simulink model "speed_controller_2017b"  (R2017b)
settings: Solver=VariableStepAuto  StartTime=0.0  StopTime=10.0  RelTol=1e-3
libraries: speedgoatlib_IO101 x2, speedgoatlib_IO106 x2, slrtlib x2
settings Model: Creator=manaka  LastModifiedBy=manaka
settings DataIOCC: ReturnWorkspaceOutputs=on
settings DebuggingCC: UnconnectedInputMsg=none  UnconnectedOutputMsg=none  UnconnectedLineMsg=none
settings ModelReferenceCC: EnableRefExpFcnMdlSchedulingChecks=off
settings SFSimCC: SimUseLocalCustomCode=on
settings RTWCC: Description=Generic Real-Time Target  RTWUseLocalCustomCode=on

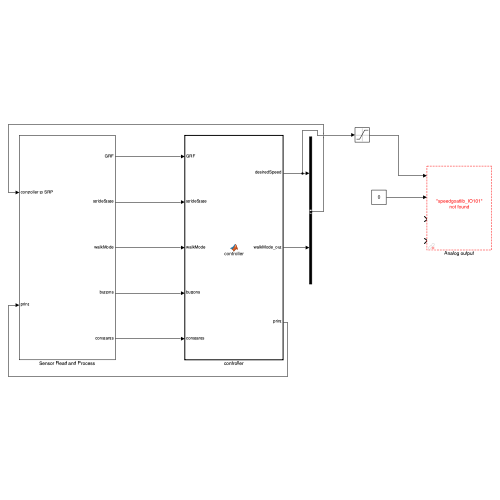
[thumbnail: Simulink's stored preview of the top-level diagram]
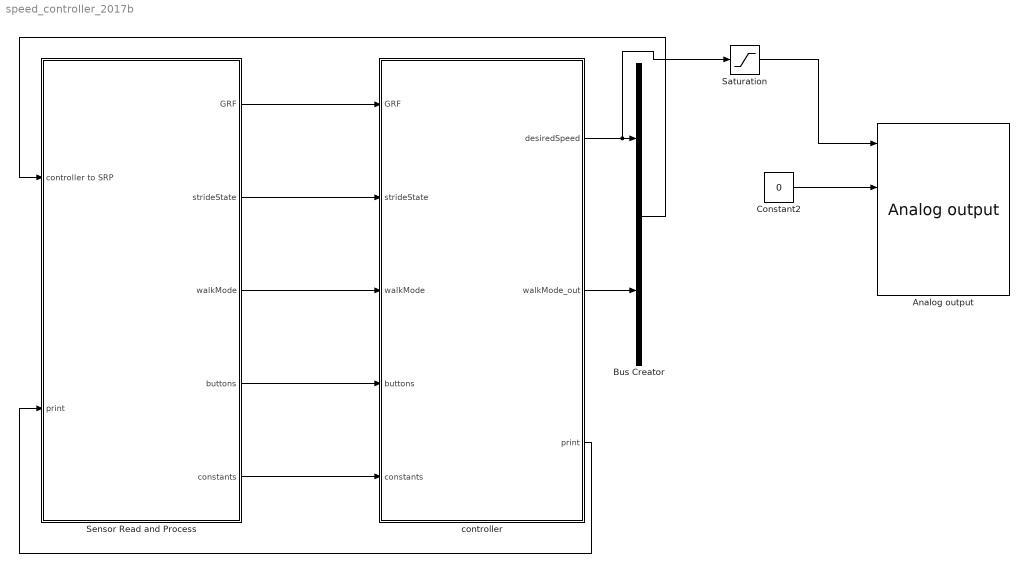
== system speed_controller_2017b ==
  Analog output : speedgoatlib_IO101/Analog output  id=1  channel=[1,2,3,4]  reset=[1,1,1,1]  initValue=[0,0,0,0]  ts=0.001  pciSlot=-1
  Bus Creator : BusCreator  Inputs=2
  Constant2 : Constant  Value=0
  Saturation : Saturate  UpperLimit=1  LowerLimit=-1
  Sensor Read and Process : Subsystem
  controller : MATLAB Function  TreatAsAtomicUnit=on
  wires:
  Sensor Read and Process/1(GRF) -> controller/1(GRF)
  Sensor Read and Process/2(strideState) -> controller/2(strideState)
  Sensor Read and Process/3(walkMode) -> controller/3(walkMode)
  Sensor Read and Process/4(buttons) -> controller/4(buttons)
  Sensor Read and Process/5(constants) -> controller/5(constants)
  Bus Creator/1 -> Sensor Read and Process/1(controller to SRP)
  controller/1(desiredSpeed) -> Saturation/1, Bus Creator/1
  controller/2(walkMode_out) -> Bus Creator/2
  controller/3(print) -> Sensor Read and Process/2(print)
  Saturation/1 -> Analog output/1
  Constant2/1 -> Analog output/2

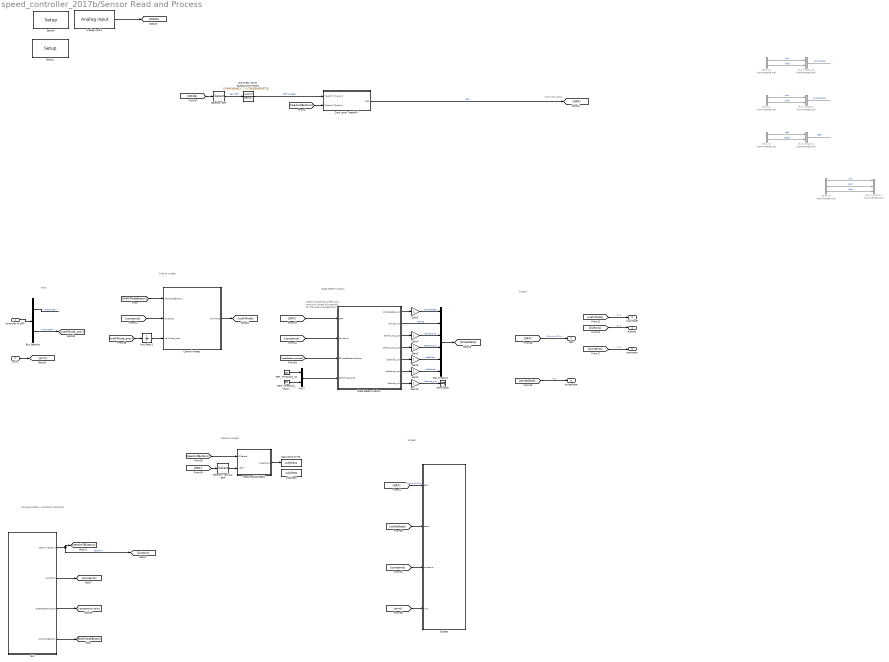
== system speed_controller_2017b/Sensor Read and Process ==
  note: Control modes
  note: Scopes
  note: Check thresholds of GRF and max/min values of threshold for stance/swing detection!
  note: State Determination
  note: GUI parameters, constants
      | & Buttons
  note: [N or Nm] 12x1
  note: Input
  note: Output
  note: Measure Weight
  controller to SRP : Inport
  print : Inport  Port=2
  "3rd Order, 25 Hz Butterworth Filter1" : DiscreteFilter  Numerator="[0.000416546139075769\t0.00124963841722731\t0.00124963841722731\t0.000416546139075769]"  Denominator="[1\t-2.68615739654814\t2.41965511096647\t-0.730165345305723]"
  Analog input3 : speedgoatlib_IO106/Analog input  id=1  channels=20  range=1  coupling=1  ts=dt  initiator=1  pciSlot=-1
  Bus Creator1 : BusCreator  Inputs=6
  Bus Creator10 : BusCreator  Commented=on  Inputs=2
  Bus Creator11 : BusCreator  Commented=on  Inputs=3
  Bus Creator3 : BusCreator  Commented=on  Inputs=2
  Bus Creator4 : BusCreator  Commented=on  Inputs=2
  Bus Selector : BusSelector  OutputSignals=prepMode,walkMode
  Control modes : MATLAB Function  TreatAsAtomicUnit=on
  Data Store Write : DataStoreWrite  DataStoreName=subjMass
  Demux : Demux  Commented=on  Outputs=2
  Demux1 : Demux  Commented=on  Outputs=2
  Demux4 : Demux  Commented=on  Outputs=2
  Demux5 : Demux  Commented=on  Outputs=3
  GRF_Threshold_Down : Constant  Value=50
  GRF_Threshold_Up : Constant  Value=100
  GUI : Subsystem
  Gain{3..5,8..10} (6 alike) : Gain
  Mux7 : Mux  Inputs=2
  Scopes : Subsystem
  Selector: GRF : Selector  InputPortWidth=20  IndexOptions=Index vector (dialog)  Indices=[1:12]  OutputSizes=1
  Selector: vertical GRF : Selector  InputPortWidth=12  IndexOptions=Index vector (dialog)  Indices=[3, 9]  OutputSizes=1
  Setup1 : speedgoatlib_IO101/Setup  group=Digital setup upper channel  id=1  pciSlot=-1  adStartChannel=1  adNumChannel=32  adCoupling=Single-ended  adRange="-10 .. 10V ==> Set  hardware DIP switches 2 5 6 9 to ON"  adAcqMode=Standard  daChannel=[1:4]  daReset=[1]  daInitValue=[0]  lowerChannel=1:8  lowerDirection=Output  lowerDIDebounce=0  lowerDOReset=[1]  lowerDOInitValues=[0]  upperChannel=1:8  upperDirection=Output  upperDIDebounce=0  upperDOReset=0  upperDOInitValues=0
  Setup4 : speedgoatlib_IO106/Setup  group=Module setup  id=1  cal=on  initiator=Initiator  pciSlot=-1  adChannel=20  adRange=+-10V  adCoupling=Single-ended
  State Determination : MATLAB Function  TreatAsAtomicUnit=on
  Terminator : Terminator
  Unit Delay1 : UnitDelay  InitialCondition=[-1;-1;-1]  SampleTime=-1  HasFrameUpgradeWarning=on
  Zero Level Treadmill : Subsystem
  measureSubjWeight : MATLAB Function  TreatAsAtomicUnit=on
  subjMass : DataStoreMemory  DataStoreName=subjMass  ReadBeforeWriteMsg=warning  WriteAfterWriteMsg=warning  WriteAfterReadMsg=warning  ShowAdditionalParam=off
  GRF : Outport  VectorParamsAs1DForOutWhenUnconnected=off
  strideState : Outport  Port=2  VectorParamsAs1DForOutWhenUnconnected=off
  walkMode : Outport  Port=3  VectorParamsAs1DForOutWhenUnconnected=off
  buttons : Outport  Port=4  VectorParamsAs1DForOutWhenUnconnected=off
  constants : Outport  Port=5  VectorParamsAs1DForOutWhenUnconnected=off
  wires:
  ? -> Demux5/1  "motorPositions rad"
  Demux5/2 -> Bus Creator11/2  "kext"
  Demux5/1 -> Bus Creator11/1  "ank"
  Demux5/3 -> Bus Creator11/3  "kflex"
  Demux/2 -> Bus Creator3/2  "knee"
  Demux/1 -> Bus Creator3/1  "ank"
  Demux4/2 -> Bus Creator10/2  "knee"
  ? -> Demux4/1
  Demux1/2 -> Bus Creator4/2  "Right"
  Bus Creator3/1 -> ?  "jointVelocity"
  ? -> Demux1/1  "GRF"
  Bus Creator4/1 -> ?  "GRF"
  ? -> Demux/1
  Demux4/1 -> Bus Creator10/1  "ank"
  Bus Creator10/1 -> ?  "jointAngle"
  Demux1/1 -> Bus Creator4/1  "Left"
  [constants] -> State Determination/2(constants)
  [IO106] -> Selector: GRF/1
  Analog input3/1 -> [IO106]
  [strideState] -> Scopes/2(state)
  [buttons] -> buttons/1  "5x1"
  [walkMode] -> walkMode/1  "1x1"
  Bus Selector/1 -> ?  "<prepMode>"
  controller to SRP/1 -> Bus Selector/1
  Control modes/1(walkMode) -> [walkMode]
  [constants] -> Control modes/2(constants)
  GUI/2("constants ") -> [constants]
  State Determination/6(pctStance_out) -> Gain9/1
  State Determination/5(pctStride_out) -> Gain8/1
  GUI/1(treadmillButtons) -> [buttons], [treadmillButtons]  "treadmill"
  [strideState] -> strideState/1  "6x1"
  State Determination/4(tStance_avg_out) -> Gain5/1
  State Determination/3(tStride_avg_out) -> Gain4/1
  State Determination/2(tStride_out) -> Bus Creator1/2  "tStride"
  State Determination/1(strideStateR_out) -> Gain3/1
  Bus Creator1/1 -> [strideState]
  GRF_Threshold_Down/1 -> Mux7/2
  GRF_Threshold_Up/1 -> Mux7/1
  Mux7/1 -> State Determination/4(GRF_Thresholds)
  [GRF] -> State Determination/1(GRF)
  Zero Level Treadmill/1(GRF) -> [GRF]  "GRF"
  "3rd Order, 25 Hz Butterworth Filter1"/1 -> Zero Level Treadmill/1(Treadmill Signals)  "GRF voltage"
  [treadmillButtons] -> Zero Level Treadmill/2(Treadmill Buttons)
  Selector: GRF/1 -> "3rd Order, 25 Hz Butterworth Filter1"/1  "Raw GRF"
  [GRF] -> GRF/1  "[N or Nm] 12x1"
  [constants] -> constants/1  "4x1"
  Bus Selector/2 -> [walkMode_prev]  "<walkMode>"
  [walkMode_prev] -> Unit Delay1/1
  Unit Delay1/1 -> Control modes/3(walkMode_prev)
  [GRF] -> Selector: vertical GRF/1
  [treadmillButtons] -> measureSubjWeight/1(BTselect)
  measureSubjWeight/1(weight_out) -> Data Store Write/1
  Selector: vertical GRF/1 -> measureSubjWeight/2(vGRF)
  Gain3/1 -> Bus Creator1/1  "strideStateR"
  Gain4/1 -> Bus Creator1/3  "tStride_avg"
  Gain5/1 -> Bus Creator1/4  "tStance_avg"
  GUI/3(resetStateVariables) -> [resetStateVariables]
  [resetStateVariables] -> State Determination/3(BTresetStateVariables)
  Gain8/1 -> Bus Creator1/5  "pctStride"
  Gain9/1 -> Bus Creator1/6  "pctStance"
  Gain10/1 -> Terminator/1  "tStance_out"
  State Determination/7(tStance_out) -> Gain10/1
  [constants] -> Scopes/3("constants ")
  print/1 -> [print]
  [print] -> Scopes/4(In14)
  [GRF] -> Scopes/1(GRF)  "[N or Nm] 12x1"
  GUI/4(WalkModeButton) -> [WalkModeButton]
  [WalkModeButton] -> Control modes/1(WalkModeButtons)

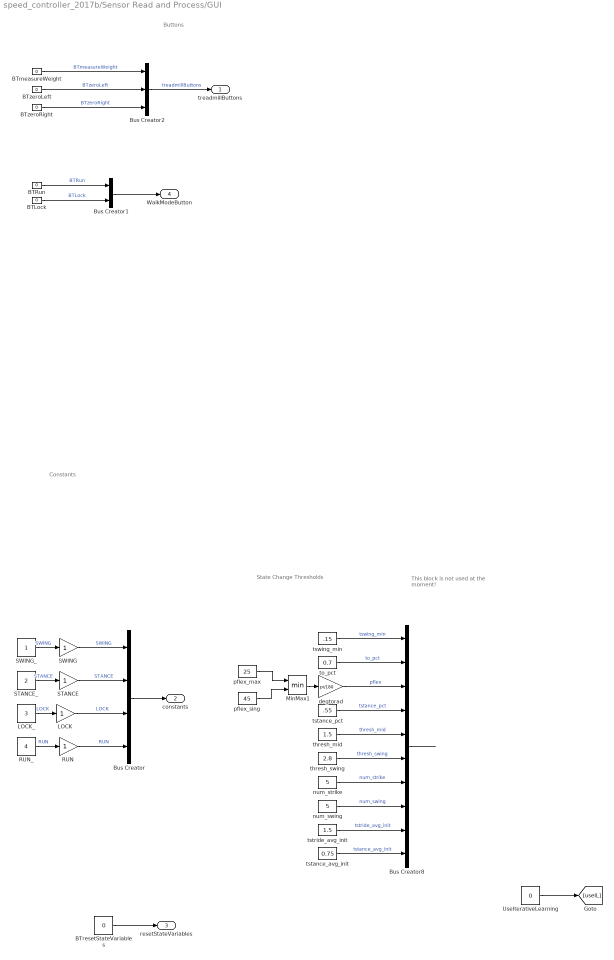
== system speed_controller_2017b/Sensor Read and Process/GUI ==
  note: Constants
  note: State Change
      | Thresholds
  note: Buttons
  note: This block is not used at the moment!
  BTLock : Constant  Tag=BTrestL  Value=0
  BTRun : Constant  Tag=BTrestL  Value=0
  BTmeasureWeight : Constant  Tag=BTrestL  Value=0
  BTresetStateVariables : Constant  Value=0
  BTzeroLeft : Constant  Tag=BTrestL  Value=0
  BTzeroRight : Constant  Tag=BTrestL  Value=0
  Bus Creator : BusCreator  Inputs=4
  Bus Creator1 : BusCreator  Inputs=2
  Bus Creator2 : BusCreator  Inputs=3
  Bus Creator8 : BusCreator  Inputs=10
  LOCK : Gain
  LOCK_ : Constant  Value=3
  MinMax1 : MinMax  Inputs=2
  RUN : Gain
  RUN_ : Constant  Value=4
  STANCE : Gain
  STANCE_ : Constant  Value=2
  SWING : Gain
  SWING_ : Constant
  UseIterativeLearning : Constant  Value=0
  degtorad : Gain  Gain=pi/180
  num_strike : Constant  Value=5
  num_swing : Constant  Value=5
  pflex_max : Constant  Value=25
  pflex_sing : Constant  Value=45
  thresh_mid : Constant  Value=1.5
  thresh_swing : Constant  Value=2.8
  to_pct : Constant  Value=0.7
  tstance_avg_init : Constant  Value=0.75
  tstance_pct : Constant  Value=.55
  tstride_avg_init : Constant  Value=1.5
  tswing_min : Constant  Value=.15
  treadmillButtons : Outport  VectorParamsAs1DForOutWhenUnconnected=off
  "constants " : Outport  Port=2  VectorParamsAs1DForOutWhenUnconnected=off
  resetStateVariables : Outport  Port=3  VectorParamsAs1DForOutWhenUnconnected=off
  WalkModeButton : Outport  Port=4
  wires:
  BTzeroLeft/1 -> Bus Creator2/2  "BTzeroLeft"
  STANCE_/1 -> STANCE/1  "STANCE"
  SWING_/1 -> SWING/1  "SWING"
  pflex_max/1 -> MinMax1/1
  thresh_swing/1 -> Bus Creator8/6  "thresh_swing"
  degtorad/1 -> Bus Creator8/3  "pflex"
  Bus Creator8/1 -> ?
  num_swing/1 -> Bus Creator8/8  "num_swing"
  pflex_sing/1 -> MinMax1/2
  num_strike/1 -> Bus Creator8/7  "num_strike"
  tstance_avg_init/1 -> Bus Creator8/10  "tstance_avg_init"
  tswing_min/1 -> Bus Creator8/1  "tswing_min"
  tstride_avg_init/1 -> Bus Creator8/9  "tstride_avg_init"
  MinMax1/1 -> degtorad/1
  tstance_pct/1 -> Bus Creator8/4  "tstance_pct"
  thresh_mid/1 -> Bus Creator8/5  "thresh_mid"
  to_pct/1 -> Bus Creator8/2  "to_pct"
  BTzeroRight/1 -> Bus Creator2/3  "BTzeroRight"
  BTmeasureWeight/1 -> Bus Creator2/1  "BTmeasureWeight"
  Bus Creator2/1 -> treadmillButtons/1  "treadmillButtons"
  SWING/1 -> Bus Creator/1  "SWING"
  STANCE/1 -> Bus Creator/2  "STANCE"
  BTresetStateVariables/1 -> resetStateVariables/1
  UseIterativeLearning/1 -> [useIL]
  Bus Creator1/1 -> WalkModeButton/1
  BTRun/1 -> Bus Creator1/1  "BTRun"
  BTLock/1 -> Bus Creator1/2  "BTLock"
  LOCK/1 -> Bus Creator/3  "LOCK"
  LOCK_/1 -> LOCK/1  "LOCK"
  RUN_/1 -> RUN/1  "RUN"
  RUN/1 -> Bus Creator/4  "RUN"
  Bus Creator/1 -> "constants "/1

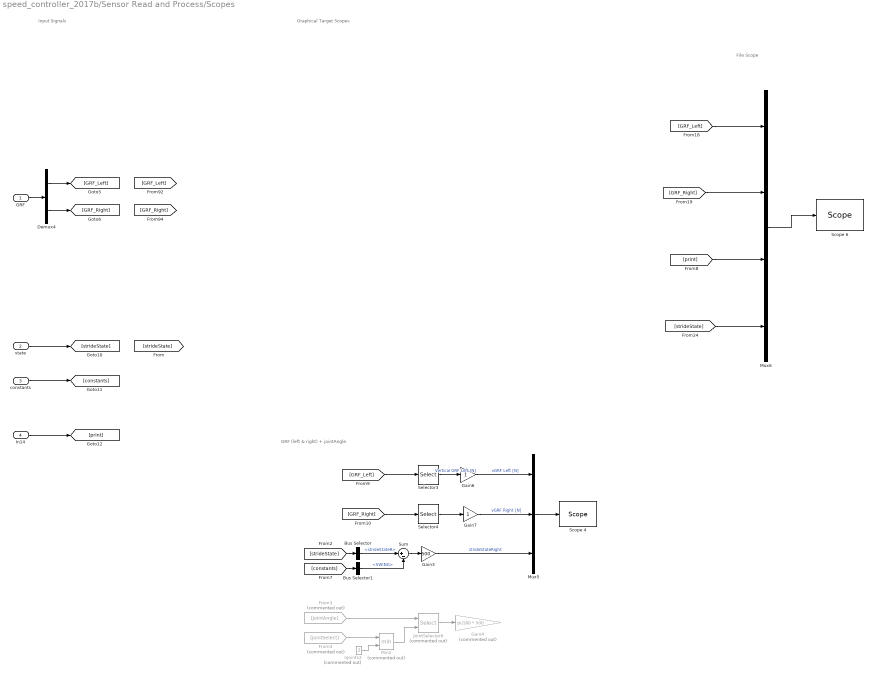
== system speed_controller_2017b/Sensor Read and Process/Scopes ==
  note: File Scope
  note: GRF (left & right) + jointAngle
  note: Graphical Target Scopes
  note: Input Signals
  GRF : Inport
  state : Inport  Port=2
  "constants " : Inport  Port=3
  In14 : Inport  Port=4
  Bus Selector : BusSelector  OutputSignals=strideStateR
  Bus Selector1 : BusSelector  OutputSignals=SWING
  Demux4 : Demux  Outputs=2
  From3 : From  Commented=on  GotoTag=jointAngle
  From4 : From  Commented=on  GotoTag=jointSelect
  Gain3 : Gain  Gain=500
  Gain4 : Gain  Commented=on  Gain=pi/180 * 500
  Gain6 : Gain
  Gain7 : Gain
  JointSelector6 : Selector  Commented=on  InputPortWidth=2  IndexOptions=Index vector (port)  Indices=[1 2]  OutputSizes=1
  Min2 : MinMax  Commented=on  Inputs=2
  Mux5 : Mux  Inputs=3
  Mux6 : Mux
  Scope 4 : slrtlib/Displays and Logging/Scope   scopeno=9  scopetype=Target  autostart=on  viewmode=Graphical rolling  formatstr='%15.6f'  grid=on  ylimits=[0,0]  nosamples=6000  noprepostsamples=0  interleave=1  triggermode=FreeRun  triggersignal=1  trigsignalfromport=off  triggerlevel=0.0  triggerslope=Either  triggerscope=1  triggersample=0  filename=data.dat  mode=Lazy  writesize=512  autorestart=off  dynamicfilemode=off  maxwritefilesize=512*1024^2
  Scope 6 : slrtlib/Displays and Logging/Scope   scopeno=5  scopetype=File  autostart=off  viewmode=Graphical redraw  formatstr='%15.6f'  grid=on  ylimits=[0,0]  nosamples=10*60*1000/2  noprepostsamples=0  interleave=2  triggermode=FreeRun  triggersignal=1  trigsignalfromport=off  triggerlevel=0.0  triggerslope=Either  triggerscope=1  triggersample=0  filename=steptest.dat  mode=Lazy  writesize=512  autorestart=off  dynamicfilemode=off  maxwritefilesize=512*1024^2
  Selector3 : Selector  InputPortWidth=6  IndexOptions=Index vector (dialog)  Indices=[3]  OutputSizes=1
  Selector4 : Selector  InputPortWidth=6  IndexOptions=Index vector (dialog)  Indices=[3]  OutputSizes=1
  Sum : Sum  Inputs=|+-
  nJoints2 : Constant  Commented=on  Value=2
  wires:
  GRF/1 -> Demux4/1
  Demux4/2 -> [GRF_Right]
  Demux4/1 -> [GRF_Left]
  Mux6/1 -> Scope 6/1
  [GRF_Left] -> Mux6/1
  Mux5/1 -> Scope 4/1
  Selector4/1 -> Gain7/1
  Selector3/1 -> Gain6/1  "Vertical GRF Left [N]"
  [GRF_Right] -> Selector4/1
  [GRF_Left] -> Selector3/1
  state/1 -> [strideState]
  [strideState] -> Bus Selector/1
  "constants "/1 -> [constants]
  [constants] -> Bus Selector1/1
  Bus Selector/1 -> Sum/1  "<strideStateR>"
  Bus Selector1/1 -> Sum/2  "<SWING>"
  Sum/1 -> Gain3/1
  Gain3/1 -> Mux5/3  "strideStateRight"
  JointSelector6/1 -> Gain4/1
  From3/1 -> JointSelector6/1
  From4/1 -> Min2/1
  nJoints2/1 -> Min2/2
  Min2/1 -> JointSelector6/2
  Gain6/1 -> Mux5/1  "vGRF Left [N]"
  Gain7/1 -> Mux5/2  "vGRF Right [N]"
  In14/1 -> [print]
  [print] -> Mux6/3
  [strideState] -> Mux6/4
  [GRF_Right] -> Mux6/2

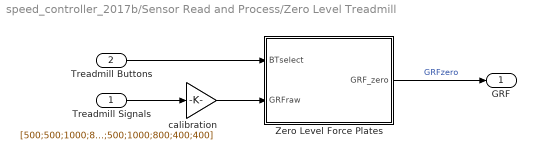
== system speed_controller_2017b/Sensor Read and Process/Zero Level Treadmill ==
  Treadmill Signals : Inport
  Treadmill Buttons : Inport  Port=2
  Zero Level Force Plates : MATLAB Function  TreatAsAtomicUnit=on
  calibration : Gain  Gain=[500;500;1000;800;400;400;500;500;1000;800;400;400]
  GRF : Outport  VectorParamsAs1DForOutWhenUnconnected=off
  wires:
  Treadmill Buttons/1 -> Zero Level Force Plates/1(BTselect)
  calibration/1 -> Zero Level Force Plates/2(GRFraw)
  Zero Level Force Plates/1(GRF_zero) -> GRF/1  "GRFzero"
  Treadmill Signals/1 -> calibration/1

== matlab function speed_controller_2017b/controller ==
  data: GRF input; desiredSpeed output; walkMode_out output; strideState input; walkMode input; buttons input; constants input; print output
function [desiredSpeed,walkMode_out,print] = controller(GRF, strideState,walkMode, buttons, constants)

% combine inputs into a single variable to be passed around
io.GRF = GRF;
io.strideState = strideState;
io.walkMode = walkMode; % port 9
io.buttons = buttons;
io.constants = constants;

outputs.desiredSpeed = 0;      % double [1x1]
outputs.walkMode = 0; 

%nodes 
NodeSpeed = [0 0.5 1.1 1.3 1.0];
NodePercent = [0 0.25 0.5 0.75 1];
speed = 0;
%currentSpeed = 0;
NodeSpeedSwing = [speed NodeSpeed(1)];
NodeSwingPercent = [0 0.5];

switch io.walkMode 
    %when walk mode is lock set the speed to 0
    case io.constants.LOCK
        outputs.desiredSpeed = 0;
    %when walk mode is run set the set the speed from nodes
    case io.constants.RUN
        if io.strideState.strideStateR_out == 1
            speed = spline(NodePercent,NodeSpeed,io.strideState.pctStride_out);
            outputs.desiredSpeed = speed;
            %currentSpeed = speed;
        elseif io.strideState.strideStateR_out == 0
            outputs.desiredSpeed = spline(NodeSpeedSwing,NodeSwingPercent,SwingPercent);           
        end
end
desiredSpeed = outputs.desiredSpeed;
walkMode_out = outputs.walkMode; 
print = 0;
end

== matlab function speed_controller_2017b/Sensor Read and Process/Control modes ==
  data: WalkModeButtons input; constants input; walkMode output; walkMode_prev input
function walkMode   = controlModes( WalkModeButtons,constants, walkMode_prev)

% prepMode
%   - constants.REST
%   - constants.SETZERO
%   - constants.WALK
% walkMode
%   - constants.ZEROTORQUE
%   - constants.TORQUE

% prepMode = [0,0,0];

% switchToTorqueMode remembers if we're trying to go to torque mode via
% button selection. This is used to prevent switching to torque mode in the
% middle of stance. 
% persistent switchToTorqueMode
% if isempty(switchToTorqueMode)
%     switchToTorqueMode = [0 0 0];
% end

% check if controller was just built - if so, start in rest mode.
% otherwise, mode determination uses previous mode as a starting point
% if all(prepMode_prev == [-1;-1;-1])
%     prepMode = [0;0;0] + constants.REST;
% else
%     prepMode = prepMode_prev;
% end

% if all(walkMode_prev == [-1;-1;-1])
%     walkMode = [0;0;0] + constants.ZEROTORQUE;
% else
%     walkMode = walkMode_prev;
% end
if walkMode_prev == -1
    walkMode = constants.LOCK;
else
    walkMode = walkMOde_prev;
end


% Change prepMode or walkMode if buttons are pressed
% if ankleButtons.BTrestAnk
%     prepMode(1) = constants.REST;
%     walkMode(1) = constants.ZEROTORQUE;
% elseif ankleButtons.BTsetzeroAnk
%     prepMode(1) = constants.SETZERO;
%     walkMode(1) = constants.ZEROTORQUE;
% elseif ankleButtons.BTwalkAnk
%     prepMode(1) = constants.WALK;
%     walkMode(1) = constants.ZEROTORQUE;
% elseif ankleButtons.BTzeroTorqueAnk
%     walkMode(1) = constants.ZEROTORQUE;
% elseif ankleButtons.BTTorqueAnk
%     switchToTorqueMode(1) = 1;
% end
% 
% if kneeButtons.BTrestKnee
%     prepMode(2:3) = constants.REST;
%     walkMode(2:3) = constants.ZEROTORQUE;
% elseif kneeButtons.BTsetzeroKnee
%     prepMode(2:3) = constants.SETZERO;
%     walkMode(2:3) = constants.ZEROTORQUE;
% elseif kneeButtons.BTwalkKnee
%     prepMode(2:3) = constants.WALK;
%     walkMode(2:3) = constants.ZEROTORQUE;
% elseif kneeButtons.BTzeroTorqueExt
%     walkMode(2:3) = constants.ZEROTORQUE;
% elseif kneeButtons.BTzeroTorqueFlx
%     walkMode(2:3) = constants.ZEROTORQUE;
% elseif kneeButtons.BTTorqueExt
%     switchToTorqueMode(2) = 1;
% elseif kneeButtons.BTTorqueFlx
%     switchToTorqueMode(3) = 1;
% end

if WalkModeButtons.BTRun
    walkMode = constants.RUN;
elseif WalkModeBUttons.BTLock
    walkMode = constants.LOCK;
end

% check switchToTorqueMode -- if any flags raised and we're in swing,
% switch that dof to torque mode and lower flag
% for dof=1:3
%     if switchToTorqueMode(dof) == 1 && strideState.strideStateR == constants.SWING
%         walkMode(dof) = constants.TORQUE;
%         switchToTorqueMode(dof) = 0;
%     end
% end

end

== matlab function speed_controller_2017b/Sensor Read and Process/State Determination ==
  data: GRF input; constants input; BTresetStateVariables input; strideStateR_out output; tStride_out output; GRF_Thresholds input; tStride_avg_out output; tStance_avg_out output; pctStride_out output; pctStance_out output; tStance_out output
function [strideStateR_out, tStride_out, tStride_avg_out, tStance_avg_out, pctStride_out, pctStance_out, tStance_out] = StateDetermination(GRF, constants, BTresetStateVariables, GRF_Thresholds)

% Constants
dt = 1/1000;                            % Sampling rate (s)
tSwing_min = 0.25;                      % Minimal swing time before new stride can be detected
tStance_min_pct = 0.62;                 % Minimum stance time in percentage of stride time before toe-off can be detected
tStance_pct = 0.4;                      % Minimum stance time in percentage of stride time to determine toe-off
tStance_vel_pct = 0.55;                 % Minimum stance time in percentage of stride time to determine toe-off for velocity crossing
AnkleAngle_max = 50;                    % Maximum plantarflexion angle before transitioning to swing
AnkleVelocity_min = 50;                 % Miniminum ankle joint velocity threshold for toe-off detection (degrees/s)
%constants = createConstants();          % See constants bus for constant values

% Unpack input signal
Fz_Right = GRF(9);                      % Vertical GRF right treadmill
Fy_Threshold_Up = GRF_Thresholds(1);    % Threshold GRF at heel strike
Fy_Threshold_Down = GRF_Thresholds(2);  % Threshold GRF at toe-off

persistent strideStateR
persistent stance
persistent tStride
persistent tStance
persistent tSwing
persistent tStride_array                % Array that contains the stride times of the last 20 strides
persistent tStance_array                % Array that contains the stance times of the last 20 strides
persistent tStride_avg
persistent tStance_avg
persistent pctStride
persistent pctStance

if isempty(strideStateR)
    strideStateR = constants.STANCE;
end
if isempty(tStride)
    tStride = 0;
end
if isempty(stance)
    stance = 0;
end
if isempty(tStance)
    tStance = 0;
end
if isempty(tSwing)
    tSwing = 0;
end
if isempty(tStride_array)
    tStride_array = 1.05 * ones(20,1);
end
if isempty(tStance_array)
    tStance_array = 0.65 * ones(20,1);
end
if isempty(tStride_avg)
    tStride_avg = 1.05;
end
if isempty(tStance_avg)
    tStance_avg = 0.65;
end
if isempty(pctStance)
    pctStance = 0;
end
if isempty(pctStride)
    pctStride = 0;
end

% Reset stride time to initial value
if BTresetStateVariables
    tStride_avg = 1.05;
    tStride_array = 1.05 * ones(20,1);
    tStance_avg = 0.65;
    tStance_array = 0.65 * ones(20,1);
end

switch strideStateR
    case constants.SWING % Switch from swing to stance
        if Fz_Right > Fy_Threshold_Up && tSwing > tSwing_min % Heel contact made
            tStride_array = [tStride; tStride_array(1:19)];     % Update array with last 20 measured stride times
            tStride = 0;                                        % Reset stride time
            tStance = 0;                                        % Reset stance time
            strideStateR = constants.STANCE;                   % Change strideStateR to staance
        end
    case constants.STANCE % Switch from stance to swing
        % Specify different checks that could be used for detection of
        % swing
        % check1 = tStance >= tStance_min_pct * tStride_avg;   	% Stance time >= 62% of stride stride time
        % check2 = AnkleJointVelocity < AnkleVelocity_min;        % Ankle joint velocity < 50 degrees/s
        % check3 = tStance > tStance_pct * tStride_avg;           % Stance time > 40% of average stride time
        % check4 = AnkleJointAngle > AnkleAngle_max;              % Ankle plantarflexion angle > 50 degrees
        % check5 = tStance > tStance_vel_pct * tStride_avg;       % Stance time > 55% of average stride time
        
        if Fz_Right < Fy_Threshold_Down % && check3 || check1 || check2 && check5 || check4 % Toe-off
            tStance_array = [tStance; tStance_array(1:19)];     % Update array with last 20 measured stance times
            tStance = 0;                                        % Reset stance time
            tSwing = 0;                                         % Reset swing time
            strideStateR = constants.SWING;                    % Change strideStateR to swing
        end
end

% Calculate average stride and stance time of last 20 strides
tStride_avg = nanmean(tStride_array);
tStance_avg = nanmean(tStance_array);

% Determine current interval as percentage of average stride time
pctStride = tStride / tStride_avg;
if pctStride > 1 % If current stride time is higher than average stride time, percentage is 100
    pctStride = 1;
end

% Determine current interval as percentage of average stance time
pctStance = tStance / tStance_avg;
% if io.constants.SWING % Percentage is zero in swing
%     pctStance = 0;    
if pctStance > 1 % If current stance time is higher than average stance time, percentage is 100
    pctStance = 1;
end

% Timers for current stride/stance/swing
tStride = tStride + dt;
tStance = tStance + dt;
tSwing = tSwing + dt;

% Create output variables
strideStateR_out = strideStateR;
tStride_out = tStride;
tStride_avg_out = tStride_avg;
tStance_avg_out = tStance_avg;
pctStride_out = pctStride;
pctStance_out = pctStance;
tStance_out = tStance;

== matlab function speed_controller_2017b/Sensor Read and Process/Zero Level Treadmill/Zero Level Force Plates ==
  data: BTselect input; GRFraw input; GRF_zero output
function GRF_zero  = fcn(BTselect,GRFraw)

persistent voltOff
if isempty(voltOff)
    voltOff = zeros(12,1);
end

% Zero level left treadmill
if BTselect.BTzeroLeft
    voltOff(1:6) = GRFraw(1:6);     % Set the offset to ccurrent voltage
end

% Zero level right treadmill
if BTselect.BTzeroRight
    voltOff(7:12) = GRFraw(7:12);   % Set the offset to ccurrent voltage
end
GRF_zero = GRFraw - voltOff;        % [Voltage] Force in Voltage

== matlab function speed_controller_2017b/Sensor Read and Process/measureSubjWeight ==
  data: BTselect input; vGRF input; weight_out output
function weight_out  = fcn(BTselect,vGRF)

persistent weight

if isempty(weight)
    weight = 0; %Voltage offset of zero
end

if BTselect.BTmeasureWeight
    weight = sum(vGRF);
end

weight_out = weight;
